simulink model "SimulationLoop"  (R2025b)
settings: Solver=VariableStepAuto  StartTime=0.0  StopTime=45  RelTol=1e-3
values from neighbouring files (symbols this model uses):
  constantsASTRA = constructConstants    [LoadSimulation.m]    (also in Variables.sldd = 1.275
                0.5
                9.80145
          ; test.m = getEntry(dataSect, 'constantsASTRA'))
  covar_vec = [accel_proc_cov; gyro_cov; mag_proc_cov]    [LoadSimulation.m]
  K = 1.470249225452176 3.4731302380274218E-15 -6.7477656839637988E-14 -5.4250108719448916E-15 6.0791134947973638E-16 1.4702492254521642 5.7131052429695607E-14 -2.5961430620246783E-14 3.3542904505295987E-16 -2.0795639349248136E-15 1.265572716793351E-14 5.0655712376772772 1.7800047037555838E-18 9.9462258665680811E-5 -3.9794016792206552E-17 2.4484525072400398E-17 -9.94622586657718E-5 -1.6450909006787953E-    [Variables.sldd]
  q = x(7:9)    [TEST1.m]
  u0 = [0; 0; constantsASTRA.g * constantsASTRA.m; 0]    [LoadSimulation.m]    (also in Variables.sldd = 0.0 0.0 12.49684875 0.0)
  x0 = zeros(18,1)    [LoadSimulation.m]    (also in Variables.sldd = 1.0 0.0 0.0 0.0 0.0 0.0 0.0 0.0 0.0 0.0 0.0 0.0 0.0 0.0 0.0 ; run_sim.m = zeros(12,1))
undefined symbols (not defined in the file or in its folder): DiscIntNeverNeededParam, F, Light, MIL, p
libraries: aerolibwind2 x1
settings Model: PacingRate=5  Creator=antho  LastModifiedBy=pplat

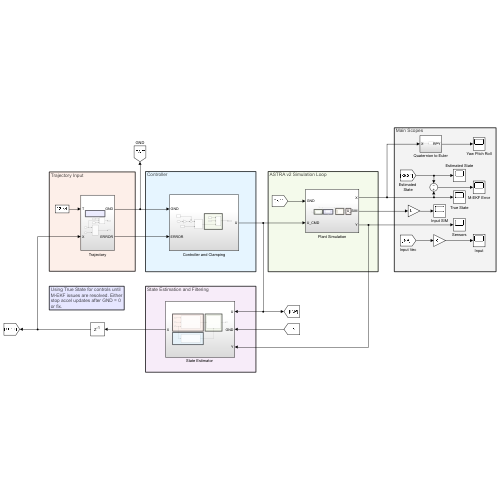
[thumbnail: Simulink's stored preview of the top-level diagram]
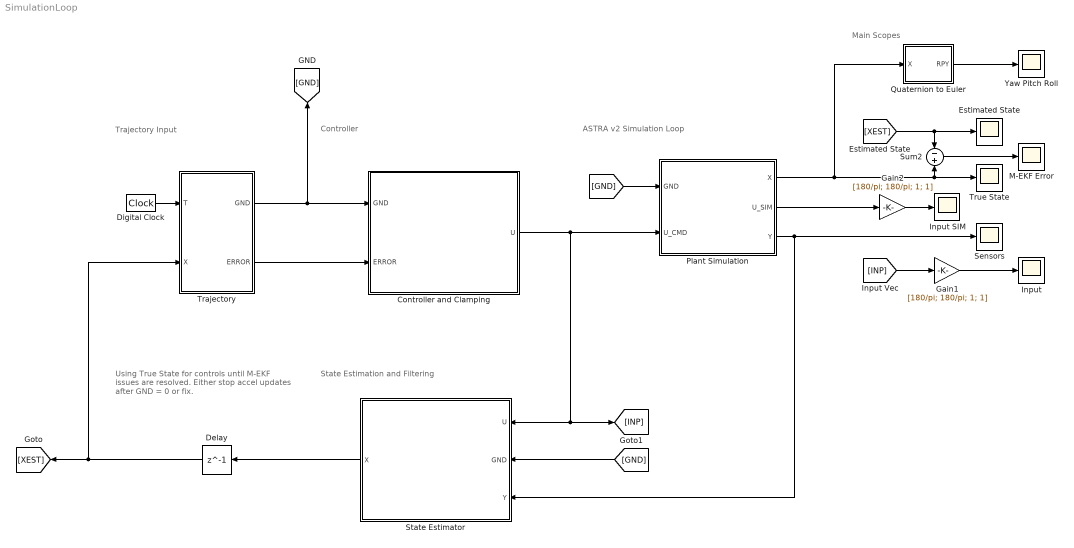
== system SimulationLoop ==
  note: Using True State for controls until
      | M-EKF issues are resolved. Either
      | stop accel updates after GND = 0
      | or fix.
  note: Main Scopes
  note: Trajectory Input
  note: State Estimation and Filtering
  note: Controller
  note: ASTRA v2 Simulation Loop
  Controller and Clamping : Subsystem
  Delay : Delay  DelayLength=1  InitialCondition=x0
  Digital Clock : DigitalClock  SampleTime=1/500
  Estimated State : Scope
      settings: ActiveDisplayYMinimum=-11.034911325111711  ActiveDisplayYMaximum=56.774891515594533
  Gain1 : Gain  Gain=[180/pi; 180/pi; 1; 1]
  Gain2 : Gain  Gain=[180/pi; 180/pi; 1; 1]
  Input : Scope
      settings: ActiveDisplayYMinimum=-2.2083284543325519  ActiveDisplayYMaximum=2.0565281030444975  DataLoggingVariableName=ScopeData6
  Input SIM : Scope
      settings: ActiveDisplayYMinimum=-10.514716193715488  ActiveDisplayYMaximum=17.393126651923364  DataLoggingVariableName=ScopeData4
  M-EKF Error : Scope
      settings: ActiveDisplayYMinimum=-0.025940833864067314  ActiveDisplayYMaximum=0.027293297670970267  DataLoggingVariableName=ScopeData2
  Plant Simulation : Subsystem
  Quaternion to Euler : Subsystem
  Sensors : Scope
      settings: ActiveDisplayYMinimum=-3.42184875911078  ActiveDisplayYMaximum=16.718947408732454  DataLoggingVariableName=ScopeData3
  "State Estimator " : Subsystem
  Sum2 : Sum  Inputs=-|+
  Trajectory : Subsystem
  True State : Scope
      settings: ActiveDisplayYMinimum=4.4434361290585729  ActiveDisplayYMaximum=5.5435067406499652
  Yaw Pitch Roll : Scope
      settings: ActiveDisplayYMinimum=-23.239291862180924  ActiveDisplayYMaximum=24.01414681727146  DataLoggingVariableName=ScopeData7
  wires:
  Digital Clock/1 -> Trajectory/1(T)
  Plant Simulation/3(Y) -> "State Estimator "/3(Y), Sensors/1
  "State Estimator "/1(X) -> Delay/1
  [XEST] -> Sum2/1, Estimated State/1
  Sum2/1 -> M-EKF Error/1
  Trajectory/2(ERROR) -> Controller and Clamping/2(ERROR)
  Controller and Clamping/1(U) -> "State Estimator "/1(U), [INP], Plant Simulation/2(U_CMD)
  Trajectory/1(GND) -> [GND], Controller and Clamping/1(GND)
  Plant Simulation/1(X) -> Quaternion to Euler/1(X), Sum2/2, True State/1
  [INP] -> Gain1/1
  Gain1/1 -> Input/1
  Delay/1 -> Trajectory/2(X), [XEST]
  Gain2/1 -> Input SIM/1
  Plant Simulation/2(U_SIM) -> Gain2/1
  Quaternion to Euler/1(RPY) -> Yaw Pitch Roll/1
  [GND] -> Plant Simulation/1(GND)
  [GND] -> "State Estimator "/2(GND)

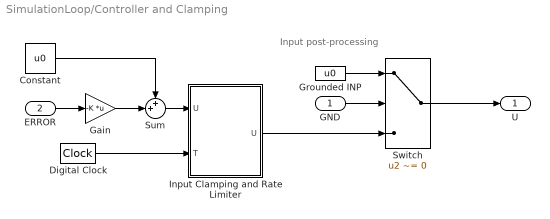
== system SimulationLoop/Controller and Clamping ==
  note: Input post-processing
  GND : Inport
  ERROR : Inport  Port=2
  Constant : Constant  Value=u0
  Digital Clock : DigitalClock  SampleTime=1/500
  Gain : Gain  Gain=-K  Multiplication=Matrix(K*u)
  Grounded INP : Constant  Value=u0
  Input Clamping and Rate Limiter : MATLAB Function  TreatAsAtomicUnit=on
  Sum : Sum  Inputs=++|
  Switch : Switch  Criteria=u2 ~= 0  SaturateOnIntegerOverflow=off  InputSameDT=off
  U : Outport
  wires:
  ERROR/1 -> Gain/1
  Digital Clock/1 -> Input Clamping and Rate Limiter/2(T)
  Input Clamping and Rate Limiter/1(U) -> Switch/3
  Switch/1 -> U/1
  Grounded INP/1 -> Switch/1
  GND/1 -> Switch/2
  Sum/1 -> Input Clamping and Rate Limiter/1("U ")
  Gain/1 -> Sum/2
  Constant/1 -> Sum/1

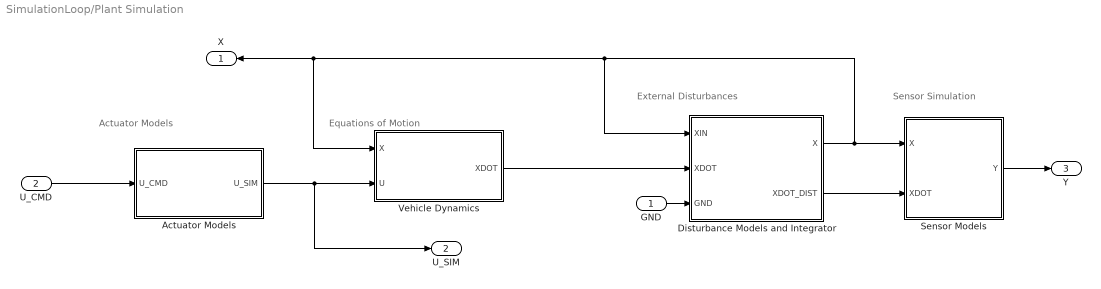
== system SimulationLoop/Plant Simulation ==
  note: Equations of Motion
  note: Actuator Models
  note: External Disturbances
  note: Sensor Simulation
  GND : Inport
  U_CMD : Inport  Port=2
  Actuator Models : Subsystem
  Disturbance Models and Integrator : Subsystem
  Sensor Models : Subsystem
  Vehicle Dynamics : Subsystem
  X : Outport
  U_SIM : Outport  Port=2
  Y : Outport  Port=3
  wires:
  U_CMD/1 -> Actuator Models/1(U_CMD)
  Vehicle Dynamics/1(XDOT) -> Disturbance Models and Integrator/2(XDOT)
  Sensor Models/1(Y) -> Y/1
  GND/1 -> Disturbance Models and Integrator/3(GND)
  Disturbance Models and Integrator/1(X) -> Disturbance Models and Integrator/1(XIN), Vehicle Dynamics/1(X), X/1, Sensor Models/1(X)
  Disturbance Models and Integrator/2(XDOT_DIST) -> Sensor Models/2(XDOT)
  Actuator Models/1(U_SIM) -> U_SIM/1, Vehicle Dynamics/2(U)

== system SimulationLoop/Quaternion to Euler ==
  X : Inport
  Quaternion to Euler : MATLAB Function  TreatAsAtomicUnit=on
  RPY : Outport
  wires:
  X/1 -> Quaternion to Euler/1(X)
  Quaternion to Euler/1(Angles) -> RPY/1

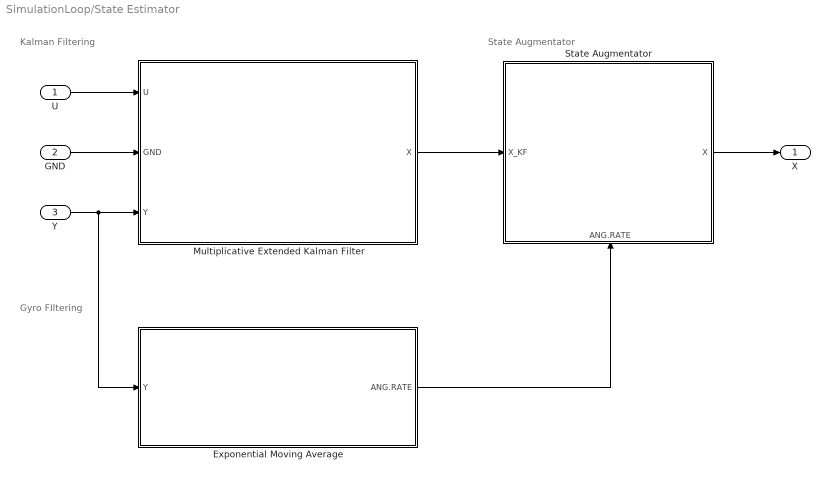
== system SimulationLoop/State Estimator  ==
  note: Gyro FIltering
  note: State Augmentator
  note: Kalman Filtering
  U : Inport
  GND : Inport  Port=2
  Y : Inport  Port=3
  "Exponential Moving Average " : Subsystem
  Multiplicative Extended Kalman Filter : Subsystem
  State Augmentator : Subsystem
      settings: PortSchema="{\"entries\":[{\"content\":{\"sides\":[{\"content\":{\"connectorIds\":[\"In1\"]},\"type\":\"ConnectorPlacement.EquallySpacedRectSide\",\"uuid\":\"bb6458aa-622a-4d42-b468-f616d6e302fe\"},{\"content\":{\"connectorIds\":[\"Out1\"],\"side\":\"RIGHT\"},\"type\":\"ConnectorPlacement.EquallySpacedRectSide\",\"uuid\":\"af8bade2-eb0a-4714-9db5-d33244eb3558\"},{\"content\":{\"side\":\"TOP\"},\"type\":\"ConnectorPlacement.EquallySpacedRectSide\",\"uuid\":\"05a7f106-e447-475e-b3b5-727cb0579a7b\"},{\"content\":{\"connectorIds\":[\"In2\"],\"side\":\"BOTTOM\"},\"type\":\"ConnectorPlacement.EquallySpacedRectSide\",\"uuid\":\"a6d44455-a42d-44f7-b37b-0d3db398c8f2\"}]},\"type\":\"ConnectorPlacement.EquallySpacedConnector\",\"uuid\":\"c6f62579-6b17-43b5-92f1-6190f0d9fd8b\"}],\"packageUris\":[\"http://schema.mathworks.com/mf0/Connector/R2020b\"],\"version\":\"1.0\"}"
  X : Outport
  wires:
  U/1 -> Multiplicative Extended Kalman Filter/1(U)
  Y/1 -> "Exponential Moving Average "/1(Y), Multiplicative Extended Kalman Filter/3(Y)
  Multiplicative Extended Kalman Filter/1(X) -> State Augmentator/1(X_KF)
  State Augmentator/1(X) -> X/1
  "Exponential Moving Average "/1(ANG.RATE) -> State Augmentator/2(ANG.RATE)
  GND/1 -> Multiplicative Extended Kalman Filter/2(GND)

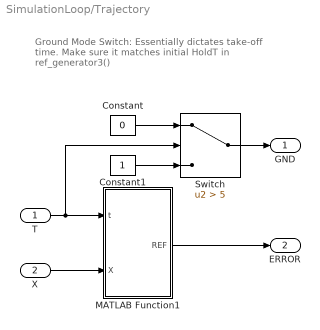
== system SimulationLoop/Trajectory ==
  note: Ground Mode Switch:
      | Essentially dictates take-off time.
      | Make sure it matches initial HoldT
      | in ref_generator3()
  T : Inport
  X : Inport  Port=2
  Constant : Constant  Value=0
  Constant1 : Constant
  MATLAB Function1 : MATLAB Function  TreatAsAtomicUnit=on
  Switch : Switch  Criteria=u2 > Threshold  Threshold=5  SaturateOnIntegerOverflow=off  InputSameDT=off
  GND : Outport
  ERROR : Outport  Port=2
  wires:
  T/1 -> Switch/2, MATLAB Function1/1(t)
  X/1 -> MATLAB Function1/2(X)
  MATLAB Function1/1(REF) -> ERROR/1
  Constant/1 -> Switch/1
  Constant1/1 -> Switch/3
  Switch/1 -> GND/1

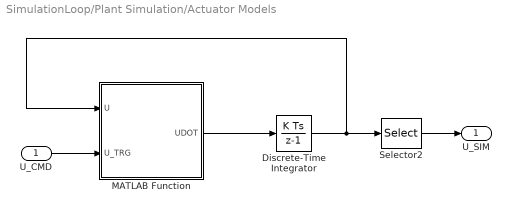
== system SimulationLoop/Plant Simulation/Actuator Models ==
  U_CMD : Inport
  Discrete-Time Integrator : DiscreteIntegrator  InitialCondition=[zeros(4,1); u0(3); 0]  SampleTime=-1  ICPrevOutput=DiscIntNeverNeededParam  ICPrevScaledInput=DiscIntNeverNeededParam
  MATLAB Function : MATLAB Function  TreatAsAtomicUnit=on
  Selector2 : Selector  InputPortWidth=6  IndexOptions=Index vector (dialog)  Indices=[1 3 5 6]  OutputSizes=1
  U_SIM : Outport
  wires:
  U_CMD/1 -> MATLAB Function/2(U_TRG)
  MATLAB Function/1(UDOT) -> Discrete-Time Integrator/1
  Discrete-Time Integrator/1 -> MATLAB Function/1(U), Selector2/1
  Selector2/1 -> U_SIM/1

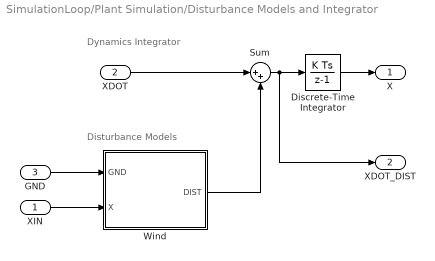
== system SimulationLoop/Plant Simulation/Disturbance Models and Integrator ==
  note: Disturbance Models
  note: Dynamics Integrator
  XIN : Inport
  XDOT : Inport  Port=2
  GND : Inport  Port=3
  Discrete-Time Integrator : DiscreteIntegrator  InitialCondition=x0  SampleTime=-1  ICPrevOutput=DiscIntNeverNeededParam  ICPrevScaledInput=DiscIntNeverNeededParam
  Sum : Sum  Inputs=|++
  Wind : Subsystem
  X : Outport
  XDOT_DIST : Outport  Port=2
  wires:
  Discrete-Time Integrator/1 -> X/1
  GND/1 -> Wind/1(GND)
  XIN/1 -> Wind/2(X)
  Wind/1(DIST) -> Sum/2
  XDOT/1 -> Sum/1
  Sum/1 -> XDOT_DIST/1, Discrete-Time Integrator/1

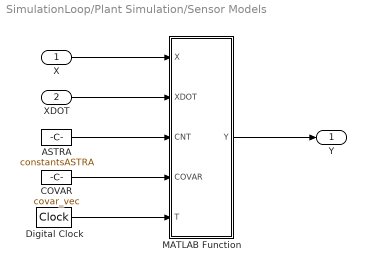
== system SimulationLoop/Plant Simulation/Sensor Models ==
  X : Inport
  XDOT : Inport  Port=2
  ASTRA : Constant  Value=constantsASTRA  OutDataTypeStr=Bus: slBus1
  COVAR : Constant  Value=covar_vec
  Digital Clock : DigitalClock  SampleTime=1/500
  MATLAB Function : MATLAB Function  TreatAsAtomicUnit=on
  Y : Outport
  wires:
  X/1 -> MATLAB Function/1(X)
  XDOT/1 -> MATLAB Function/2(XDOT)
  ASTRA/1 -> MATLAB Function/3(CNT)
  COVAR/1 -> MATLAB Function/4(COVAR)
  Digital Clock/1 -> MATLAB Function/5(T)
  MATLAB Function/1(Y) -> Y/1

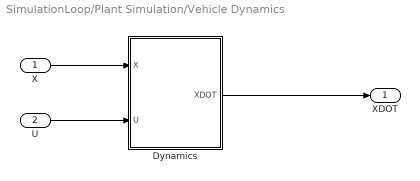
== system SimulationLoop/Plant Simulation/Vehicle Dynamics ==
  X : Inport
  U : Inport  Port=2
  Dynamics : MATLAB Function  TreatAsAtomicUnit=on
  XDOT : Outport
  wires:
  Dynamics/1(XDOT) -> XDOT/1
  U/1 -> Dynamics/2(U)
  X/1 -> Dynamics/1(X)

== system SimulationLoop/State Estimator /Exponential Moving Average  ==
  Y : Inport
  EMA Filter : MATLAB Function  TreatAsAtomicUnit=on
  ANG.RATE : Outport
  wires:
  Y/1 -> EMA Filter/1(Y)
  EMA Filter/1(EMA_G) -> ANG.RATE/1

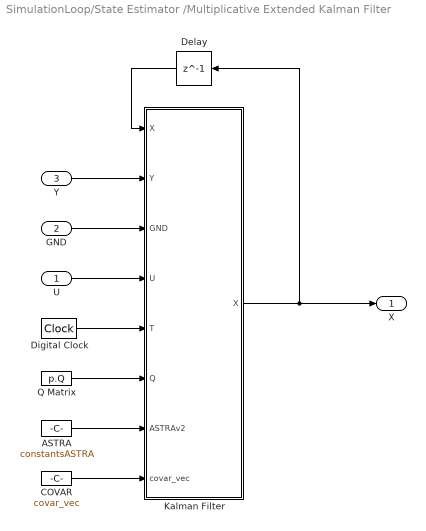
== system SimulationLoop/State Estimator /Multiplicative Extended Kalman Filter ==
  U : Inport
  GND : Inport  Port=2
  Y : Inport  Port=3
  ASTRA : Constant  Value=constantsASTRA  OutDataTypeStr=Bus: slBus1
  COVAR : Constant  Value=covar_vec
  Delay : Delay  DelayLength=1  InitialCondition=[x0(1:9); x0(13:15)]
  Digital Clock : DigitalClock  SampleTime=1/500
  Kalman Filter : MATLAB Function  TreatAsAtomicUnit=on
  Q Matrix : Constant  Value=p.Q
  X : Outport
  wires:
  Digital Clock/1 -> Kalman Filter/5(T)
  Kalman Filter/1(X) -> Delay/1, X/1
  U/1 -> Kalman Filter/4(U)
  COVAR/1 -> Kalman Filter/8(covar_vec)
  Y/1 -> Kalman Filter/2(Y)
  Delay/1 -> Kalman Filter/1("X ")
  ASTRA/1 -> Kalman Filter/7(ASTRAv2)
  Q Matrix/1 -> Kalman Filter/6(Q)
  GND/1 -> Kalman Filter/3(GND)

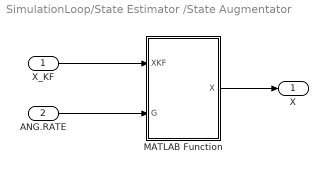
== system SimulationLoop/State Estimator /State Augmentator ==
  X_KF : Inport
  ANG.RATE : Inport  Port=2
  MATLAB Function : MATLAB Function  TreatAsAtomicUnit=on
  X : Outport
  wires:
  X_KF/1 -> MATLAB Function/1(XKF)
  MATLAB Function/1(X) -> X/1
  ANG.RATE/1 -> MATLAB Function/2(G)

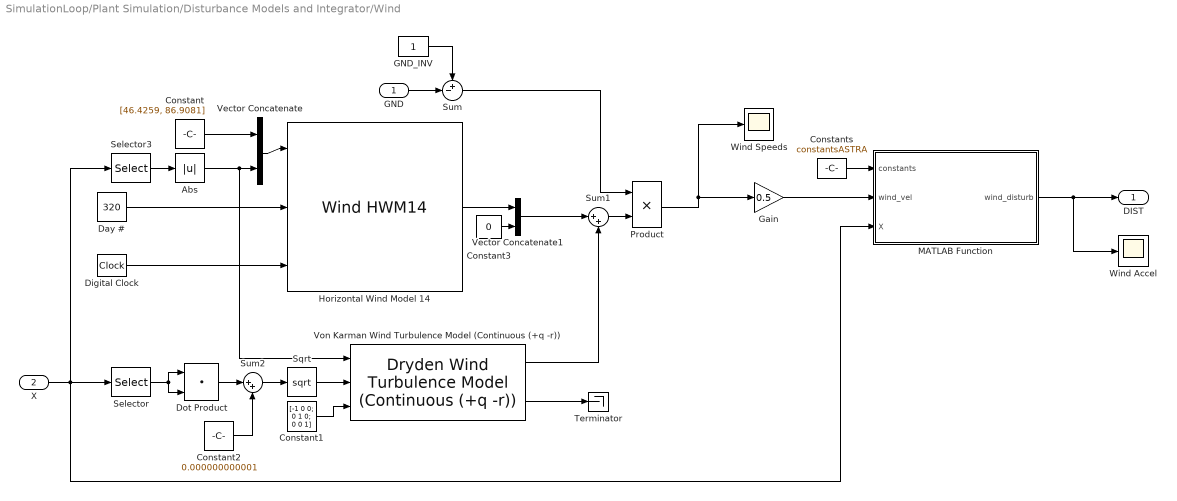
== system SimulationLoop/Plant Simulation/Disturbance Models and Integrator/Wind ==
  GND : Inport
  X : Inport  Port=2
  Abs : Abs  SaturateOnIntegerOverflow=off
  Constant : Constant  Value=[46.4259, 86.9081]
  Constant1 : Constant  Value=[-1 0 0; 0 1 0; 0 0 1]
  Constant2 : Constant  Value=0.000000000001
  Constant3 : Constant  Value=0
  Constants : Constant  Value=constantsASTRA  OutDataTypeStr=Bus: slBus1
  Day # : Constant  Value=320
  Digital Clock : DigitalClock  SampleTime=1/500
  Dot Product : DotProduct  OutDataTypeStr=Inherit: Inherit via internal rule
  GND_INV : Constant
  Gain : Gain  Gain=0.5
  Horizontal Wind Model 14 : WindHWM14
  MATLAB Function : MATLAB Function  TreatAsAtomicUnit=on
  Product : Product
  Selector : Selector  InputPortWidth=15  IndexOptions=Index vector (dialog)  Indices=[7 9]  OutputSizes=1
  Selector3 : Selector  InputPortWidth=15  IndexOptions=Index vector (dialog)  Indices=6  OutputSizes=1
  Sqrt : Sqrt
  Sum : Sum  Inputs=+-|
  Sum1 : Sum  Inputs=|++
  Sum2 : Sum  Inputs=|++
  Terminator : Terminator
  Vector Concatenate : Concatenate
  Vector Concatenate1 : Concatenate
  Von Karman Wind Turbulence Model (Continuous (+q -r)) : aerolibwind2/Dryden Wind Turbulence Model  (Continuous (+q -r))  units=Metric (MKS)  spec=MIL-F-8785C  model=Continuous Von Karman (+q -r)  W20=15  Wdeg=0  TurbProb=10^-2 - Light  L_high=762  Wingspan=10  ts=0.1  Seed=[23341 23342 23343 23344]  T_on=on
      settings: LibrarySourceBlock=|
      | aerolibwind2/Von Karman Wind Turbulence Model
      | (Continuous (+q -r))
  Wind Accel : Scope
      settings: ActiveDisplayYMinimum=-1.348262134901125  ActiveDisplayYMaximum=3.72316275685178  DataLoggingVariableName=ScopeData5
  Wind Speeds : Scope
      settings: ActiveDisplayYMinimum=-4.3320011628089352  ActiveDisplayYMaximum=5.2248552561557382  DataLoggingVariableName=ScopeData5
  DIST : Outport
  wires:
  Digital Clock/1 -> Horizontal Wind Model 14/3
  Day #/1 -> Horizontal Wind Model 14/2
  MATLAB Function/1(wind_disturb) -> Wind Accel/1, DIST/1
  Vector Concatenate/1 -> Horizontal Wind Model 14/1
  Selector3/1 -> Abs/1
  Constant/1 -> Vector Concatenate/1
  GND/1 -> Sum/2
  Sum/1 -> Product/1
  GND_INV/1 -> Sum/1
  Horizontal Wind Model 14/1 -> Vector Concatenate1/1
  Constants/1 -> MATLAB Function/1(constants)
  Selector/1 -> Dot Product/1, Dot Product/2
  Sqrt/1 -> Von Karman Wind Turbulence Model (Continuous (+q -r))/2
  Von Karman Wind Turbulence Model (Continuous (+q -r))/1 -> Sum1/2
  Sum1/1 -> Product/2
  Constant1/1 -> Von Karman Wind Turbulence Model (Continuous (+q -r))/3
  Sum2/1 -> Sqrt/1
  Dot Product/1 -> Sum2/1
  Constant2/1 -> Sum2/2
  X/1 -> MATLAB Function/3(X), Selector/1, Selector3/1
  Abs/1 -> Von Karman Wind Turbulence Model (Continuous (+q -r))/1, Vector Concatenate/2
  Product/1 -> Gain/1, Wind Speeds/1
  Vector Concatenate1/1 -> Sum1/1
  Constant3/1 -> Vector Concatenate1/2
  Von Karman Wind Turbulence Model (Continuous (+q -r))/2 -> Terminator/1
  Gain/1 -> MATLAB Function/2(wind_vel)

== matlab function SimulationLoop/Plant Simulation/Vehicle Dynamics/Dynamics ==
  data: X input; XDOT output; U input
function XDOT = Dynamics(X, U)

XDOT = nominalDynamics(X, U);

== matlab function SimulationLoop/Controller and Clamping/Input Clamping and Rate Limiter ==
  data: U input; U output; T input
function U = INPUTFCN(U, T)

    U = inputfcn3(U, T)';

== matlab function SimulationLoop/Trajectory/MATLAB Function1 ==
  data: t input; X input; REF output
function REF = RefSignal(t, X)

REF = ref_generator3(X, t);

== matlab function SimulationLoop/Plant Simulation/Sensor Models/MATLAB Function ==
  data: X input; Y output; XDOT input; CNT input; COVAR input; T input
function Y = Sensors(X, XDOT, CNT, COVAR, T)

Y = SensorSimulation(X, XDOT, CNT, COVAR, T);

== matlab function SimulationLoop/State Estimator /Multiplicative Extended Kalman Filter/Kalman Filter ==
  data: X input; Y input; GND input; X output; U input; T input; Q input; ASTRAv2 input; covar_vec input
function X = MEKF(X, Y, GND, U, T, Q, ASTRAv2, covar_vec)

    % Measure simulation timestep
    persistent dt lastT
    if isempty(dt)
        dt = 0;
        lastT = 0;
    end
    dt = T - lastT;
    lastT = T;

    X = EstimateStateFCN(X, U, ASTRAv2, Y, covar_vec, dt, Q, GND);

== matlab function SimulationLoop/Plant Simulation/Disturbance Models and Integrator/Wind/MATLAB Function ==
  data: constants input; wind_vel input; X input; wind_disturb output
function wind_disturb = wind_sim(constants, wind_vel, X)

wind_disturb = wind(constants, wind_vel, X);

== matlab function SimulationLoop/Plant Simulation/Actuator Models/MATLAB Function ==
  data: U input; UDOT output; U_TRG input
function UDOT = Actuators(U, U_TRG)

    UDOT = ActuatorDynamics(U, U_TRG);
end

== matlab function SimulationLoop/Quaternion to Euler/Quaternion to Euler ==
  data: X input; Angles output
function Angles = q2eul(X)

% Complete quaternion
qv = X(1:3);
q0 = sqrt(abs(1 - qv'*qv));
q = [q0; qv];

% Quaternion to Euler Angles
Roll = atan2(2*(q(1) * q(2) + q(3) * q(4)), 1 - 2*(q(2)^2 + q(3)^2));
Pitch = asin(2*(q(1) * q(3) - q(4) * q(2)));
Yaw = atan2(2*(q(1) * q(4) + q(2) * q(3)), 1 - 2*(q(3)^2 + q(4)^2));

% Angle Vector
Angles = [Roll; Pitch; Yaw] * 180/pi;

== matlab function SimulationLoop/State Estimator /Exponential Moving Average /EMA Filter ==
  data: Y input; EMA_G output
function EMA_G = EMA_Gyros(Y)

% Extract Gyros
gyros = Y(4:6);

% Exponential Moving Avg Step
EMA_G = ExpMovingAvg(gyros);

== matlab function SimulationLoop/State Estimator /State Augmentator/MATLAB Function ==
  data: XKF input; X output; G input
function X = StateAUG(XKF, G)

X = [XKF(1:9); G; XKF(10:12)];
